simulink model "modelofisicocompletoo"  (R2020a)
settings: Solver=FixedStepAuto  StartTime=0.0  StopTime=inf  FixedStep=0.5e-3  MaxStep=1e-3  RelTol=1e-3
PreLoadFcn:
  | Boat_State = Simulink.Signal;
  | Boat_State.DataType = 'double';
  | Boat_State.SamplingMode = 'Sample based';
  | Boat_State.InitialValue = '[6; 5; 10; 6;  3; 4]';
  | Boat_State.StorageClass = 'ExportedGlobal';
  | Boat_State.Complexity = 'real';
  | Boat_State.Description = 'dsm_description';
undefined symbols (not defined in the file): bac, baiz, bcx, bcy, Beqtran, Bheqd, bw, DiscIntNeverNeededParam, g, Kcy, ksac, ksaiz, ksiac, ksiaiz, Kw, lh0, Meq, Mheq, Rd, Rr, rt, rtd, xl0, xt0, yl0, yt0
libraries: simulink x13, powerlib_meascontrol x4, opclib x4, vrlib x2, dspswit3 x1
(part 2 of 2)

== stateflow chart modelofisicocompletoo/Level1 ==
  state EmergencyMode
  state OFF
  state Sim_pulsadorONOFF1
  state Sim_pulsadorONOFF
  state ON
    state Level1
      state Deegre_Balancer [parallel]
        settings: executionOrder=1
        state OFF
          entry: balancer =0
        state Sim_pulsador
        state Sim_pulsador1
        state ON
          entry: balancer =1
        (default) -> ON.Level1.Deegre_Balancer.OFF
        Sim_pulsador -> ON.Level1.Deegre_Balancer.OFF : [balance_switch==0]
        ON.Level1.Deegre_Balancer.OFF -> ON.Level1.Deegre_Balancer.Sim_pulsador1 : [balance_switch==1]
        ON.Level1.Deegre_Balancer.ON -> Sim_pulsador : [balance_switch==1]
        ON.Level1.Deegre_Balancer.Sim_pulsador1 -> ON.Level1.Deegre_Balancer.ON : [balance_switch==0]
      state Operation_mode [parallel]
        settings: executionOrder=2
        state Automatic
          state Waiting_for_mode
          state Double_cycle
            entry: flag_semiauto = 1;
            flag_end_traj=0;
            flag_send_traj = 0;
            reset_going=0;
            reset_down=0;
            mode_balance = 1;
            state To_boat
              entry:  [vyt,vxt,xend,vx_end,vy_end,len,len2,nx_state] = gen_traj_boat(Boat_State,xl0,yl0,container_x_position,Load_state,Total_mass);
              vx_t=vxt; vy_t=vyt;vxend_t=vx_end;vyend_t=vy_end;len_out=len;len_out2 = len2;Boat_State=nx_state;
              state Go
                entry:
                flag_send_traj = 1;
                reset_going=1;
              state Go_down
                entry:
                flag_send_traj = 1;
                flag_end_traj =1;
                reset_down =1;
              state Finished
                entry:
                flag_end_traj=0;
                flag_send_traj = 0;
              (default) -> ON.Level1.Operation_mode.Automatic.Double_cycle.To_boat.Go
              ON.Level1.Operation_mode.Automatic.Double_cycle.To_boat.Go_down -> ON.Level1.Operation_mode.Automatic.Double_cycle.To_boat.Finished : [flag_finished_taj==1]
              ON.Level1.Operation_mode.Automatic.Double_cycle.To_boat.Go -> ON.Level1.Operation_mode.Automatic.Double_cycle.To_boat.Go_down : [(abs(xend-xl0) <= 0.05) && (theta_amp <= 0.5)]
            state container_to_container
              entry: mode_balance=1;
              [vyt,vxt,xend,vx_end,vy_end,len,len2,nx_state] = gen_traj_cont_cont(Boat_State,xl0,yl0,container_x_position,Load_state,Total_mass);
              vx_t=vxt; vy_t=vyt;vxend_t=vx_end;vyend_t=vy_end;len_out=len;len_out2 = len2;Boat_State=nx_state;
              state Go_down
                entry:
                flag_send_traj = 1;
                flag_end_traj=1;
                reset_down =0;
              state Go
                entry:
                flag_send_traj = 1;
                reset_going=0;
              state Finished1
                entry:
                flag_end_traj=0;
                flag_send_traj = 0;
              (default) -> ON.Level1.Operation_mode.Automatic.Double_cycle.container_to_container.Go
              ON.Level1.Operation_mode.Automatic.Double_cycle.container_to_container.Go -> ON.Level1.Operation_mode.Automatic.Double_cycle.container_to_container.Go_down : [(abs(xend-xl0) <= 0.001) && (theta_amp <= 0.5)]
              ON.Level1.Operation_mode.Automatic.Double_cycle.container_to_container.Go_down -> Finished1 : [flag_finished_taj==1]
            state To_dock
              entry:mode_balance=0;
              [vyt,vxt,xend,vx_end,vy_end,len,len2,nx_state] = gen_traj_dock(Boat_State,xl0,yl0,1,Load_state,Total_mass);
              vx_t=vxt; vy_t=vyt;vxend_t=vx_end;vyend_t=vy_end; len_out=len; len_out2 = len2;Boat_State=nx_state;
              state Go_down
                entry:
                flag_send_traj = 1;
                flag_end_traj=1;
                reset_down =1;
              state Go
                entry:
                flag_send_traj = 1;
                reset_going=1;
              state Finished
                entry:
                flag_semiauto=0;
              (default) -> ON.Level1.Operation_mode.Automatic.Double_cycle.To_dock.Go
              ON.Level1.Operation_mode.Automatic.Double_cycle.To_dock.Go -> ON.Level1.Operation_mode.Automatic.Double_cycle.To_dock.Go_down : [(abs(xend-xl0) <= 1.5) && (theta_amp <= 1.0)]
              ON.Level1.Operation_mode.Automatic.Double_cycle.To_dock.Go_down -> ON.Level1.Operation_mode.Automatic.Double_cycle.To_dock.Finished : [flag_finished_taj==1]
            (default) -> ON.Level1.Operation_mode.Automatic.Double_cycle.To_boat
            ON.Level1.Operation_mode.Automatic.Double_cycle.To_boat.Finished -> container_to_container
            Finished1 -> ON.Level1.Operation_mode.Automatic.Double_cycle.To_dock
          state Simple_cycle
            entry: flag_semiauto = 1;
            flag_end_traj=0;
            flag_send_traj = 0;
            mode_balance = 1;
            state To_boat
              entry: flag_gen_traj = 1;
              [vyt,vxt,xend,vx_end,vy_end,len,len2,nx_state] = gen_traj_boat(Boat_State,xl0,yl0,container_x_position,Load_state,Total_mass);
              vx_t=vxt; vy_t=vyt;vxend_t=vx_end;vyend_t=vy_end;len_out=len;len_out2 = len2;Boat_State=nx_state;
              state Go
                entry:
                flag_send_traj = 1;
                reset_going =0;
              state Go_down
                entry:
                flag_send_traj = 1;
                flag_end_traj =1;
                reset_down=0;
              state Finished
                entry:
                flag_end_traj=0;
                flag_send_traj = 0;
              (default) -> ON.Level1.Operation_mode.Automatic.Simple_cycle.To_boat.Go
              ON.Level1.Operation_mode.Automatic.Simple_cycle.To_boat.Go_down -> ON.Level1.Operation_mode.Automatic.Simple_cycle.To_boat.Finished : [flag_finished_taj==1]
              ON.Level1.Operation_mode.Automatic.Simple_cycle.To_boat.Go -> ON.Level1.Operation_mode.Automatic.Simple_cycle.To_boat.Go_down : [(abs(xend-xl0) <= 0.05) && (theta_amp <= 0.5)]
            state To_dock
              entry:mode_balance=1;
              [vyt,vxt,xend,vx_end,vy_end,len,len2,nx_state] = gen_traj_dock(Boat_State,xl0,yl0,1,Load_state,Total_mass);
              vx_t=vxt; vy_t=vyt;vxend_t=vx_end;vyend_t=vy_end; len_out=len; len_out2 = len2;Boat_State=nx_state;
              state Go_down
                entry:
                flag_send_traj = 1;
                flag_end_traj=1;
                reset_down =1;
              state Go
                entry:
                flag_send_traj = 1;
                reset_going=1;
              state Finished
                entry:
                flag_semiauto=0;
              (default) -> ON.Level1.Operation_mode.Automatic.Simple_cycle.To_dock.Go
              ON.Level1.Operation_mode.Automatic.Simple_cycle.To_dock.Go -> ON.Level1.Operation_mode.Automatic.Simple_cycle.To_dock.Go_down : [(abs(xend-xl0) <= 0.001) && (theta_amp <= 1.0)]
              ON.Level1.Operation_mode.Automatic.Simple_cycle.To_dock.Go_down -> ON.Level1.Operation_mode.Automatic.Simple_cycle.To_dock.Finished : [flag_finished_taj==1]
            (default) -> ON.Level1.Operation_mode.Automatic.Simple_cycle.To_boat
          (default) -> Waiting_for_mode
          Waiting_for_mode -> Double_cycle [order 1] : [Automatic_mode==1]
          Waiting_for_mode -> Simple_cycle [order 2] : [Automatic_mode==0]
        state Manual
          entry:
          flag_semiauto = 0;
          limit_going_down=0;
          limit_vxt_down=0;
          state Operator_handling_load
            state Taking_down
              entry: limit_vxt_down=1;
              state On_air
              state Contact_floor
                entry: limit_going_down =1;
                mode_balance = 0;
              (default) -> ON.Level1.Operation_mode.Manual.Operator_handling_load.Taking_down.On_air
              ON.Level1.Operation_mode.Manual.Operator_handling_load.Taking_down.On_air -> ON.Level1.Operation_mode.Manual.Operator_handling_load.Taking_down.Contact_floor : [Fw<=0.0001]
            state Taking_off
              state On_floor
              state On_air
                entry: limit_going_down =0;
                exit:limit_vxt_down=0;
                mode_balance = 1;
              (default) -> On_floor
              On_floor -> ON.Level1.Operation_mode.Manual.Operator_handling_load.Taking_off.On_air : [Stable_FW_flag]
            (default) -> ON.Level1.Operation_mode.Manual.Operator_handling_load.Taking_down
            ON.Level1.Operation_mode.Manual.Operator_handling_load.Taking_down.Contact_floor -> Taking_off
          state Operator_handling_unload
            entry: limit_vxt_down=1;
            state Taking_down
              state On_air
              state Contact_floor
                entry: limit_going_down =1;
                mode_balance = 0;
              (default) -> ON.Level1.Operation_mode.Manual.Operator_handling_unload.Taking_down.On_air
              ON.Level1.Operation_mode.Manual.Operator_handling_unload.Taking_down.On_air -> ON.Level1.Operation_mode.Manual.Operator_handling_unload.Taking_down.Contact_floor : [Fw<=0.0001]
            state Unloading
              state On_floor_wait_unload
                entry:
                reset_calc_mass =1
              state Transiton
                entry:
                Stable_FW_flag=false
              state On_air
                entry: limit_going_down =0;
                mode_balance = 1;
                exit: limit_vxt_down=0;
              (default) -> On_floor_wait_unload
              On_floor_wait_unload -> Transiton : [Load_state==0]
              Transiton -> ON.Level1.Operation_mode.Manual.Operator_handling_unload.Unloading.On_air : [Stable_FW_flag]
            (default) -> ON.Level1.Operation_mode.Manual.Operator_handling_unload.Taking_down
            ON.Level1.Operation_mode.Manual.Operator_handling_unload.Taking_down.Contact_floor -> Unloading
          (default) -> Operator_handling_load
        state Sim_pulsador_aut
        state Sim_pulsador_man
        (default) -> Manual
        Manual -> Sim_pulsador_aut : [switch_mode==1]
        Sim_pulsador_aut -> Automatic : [switch_mode==0]
        Automatic -> Sim_pulsador_man : [switch_mode==1]
        ON.Level1.Operation_mode.Automatic.Simple_cycle.To_boat.Finished -> Operator_handling_unload : [Automatic_mode==0]
        Sim_pulsador_man -> Manual : [switch_mode==0]
        ON.Level1.Operation_mode.Manual.Operator_handling_unload.Unloading.On_air -> ON.Level1.Operation_mode.Automatic.Simple_cycle.To_dock : [flag_finished_taj==1 && Automatic_mode==0]
      state Load [parallel]
        settings: executionOrder=3
        state not_loaded
          entry: Load_state = 0;
          Total_mass = 15000
          flag_add_random_mass =0;
        state Sim_pulsador2
        state Sim_pulsador1
        state loaded
          entry: Load_state=1;
          flag_add_random_mass =1;
          random_mass = get_rand_mass()
        (default) -> not_loaded
        not_loaded -> ON.Level1.Load.Sim_pulsador1 : [twistlock==1]
        Sim_pulsador2 -> not_loaded : [twistlock==0]
        loaded -> Sim_pulsador2 : [twistlock==1]
        ON.Level1.Load.Sim_pulsador1 -> loaded : [twistlock==0]
  ON -> EmergencyMode [order 2] : [flag_enable_breaks]
  EmergencyMode -> ON : [flag_enable_level1]
  Sim_pulsadorONOFF1 -> OFF : [switch_energy==0]
  OFF -> Sim_pulsadorONOFF : [switch_energy==1]
  ON -> Sim_pulsadorONOFF1 [order 1] : [switch_energy==1]
  (default) -> ON
  Sim_pulsadorONOFF -> ON : [switch_energy==0]
  data: estado_barco function_input; posx_init function_input; posy_init function_input; posx_end function_input; twistlocks function_input; vdyt function_output; vdxt function_output; x_end function_output; vxt_end function_output; vyt_end function_output; ml function_input; lenght function_output; lenght2 function_output; next_state function_output; estado_barco function_input; posx_init function_input; posy_init function_input; posx_end function_input; twistlocks function_input; vdyt function_output; vdxt function_output; x_end function_output; vxt_end function_output; vyt_end function_output; ml function_input; lenght function_output; lenght2 function_output; next_state function_output; estado_barco function_input; posx_init function_input; posy_init function_input; posx_end function_input; twistlocks function_input; vdyt function_output; vdxt function_output; x_end function_output; vxt_end function_output; vyt_end function_output; ml function_input; lenght function_output; lenght2 function_output; next_state function_output; estado_barco function_input; posx_init function_input; posy_init function_input; posx_end function_input; twistlocks function_input; vdyt function_output; vdxt function_output; x_end function_output; vxt_end function_output; vyt_end function_output; ml function_input; lenght function_output; lenght2 function_output; next_state function_output; estado_barco function_input; posx_init function_input; posy_init function_input; posx_end function_input; twistlocks function_input; vdyt function_output; vdxt function_output; x_end function_output; vxt_end function_output; vyt_end function_output; ml function_input; lenght function_output; lenght2 function_output; next_state function_output; rand_mass function_output; xl0 input; switch_mode input; flag_semiauto output; flag_send_traj output; xend local double; flag_end_traj output; vyt local size=20000000,1; vxt local size=20000000,1; vy_end local size=20000000,1; vx_end local size=20000000,1; balance_switch input; switch_energy input; flag_finished_taj input; vyend_t output size=20000000,1; vy_t output size=20000000,1; vxend_t output size=20000000,1; vx_t output size=20000000,1; len_out output; len local; reset_down output; reset_going output; Boat_State data_store_memory; nx_state local double size=6,1 =[0; 0; 0; 0; 0; 0]; len2 local; len_out2 output; limit_vxt_down output; balancer output; mode_balance output; twistlock input; Load_state data_store_memory; limit_going_down output; Stable_FW_flag data_store_memory; Total_mass data_store_memory; container_x_position data_store_memory; flag_add_random_mass output; random_mass output; reset_calc_mass output; flag_enable_level1 input; flag_enable_breaks input; Fw input; theta_amp input; yl0 input; Automatic_mode data_store_memory; flag_gen_traj output
  function [vdyt,vdxt,x_end,vxt_end,vyt_end,lenght,lenght2,next_state] = gen_traj_boat(estado_barco,posx_init,posy_init,posx_end,twistlocks,ml):
    | function [vdyt,vdxt,x_end,vxt_end,vyt_end,lenght,lenght2,next_state] = gen_traj_boat(estado_barco,posx_init,posy_init,posx_end,twistlocks,ml)
    | coder.extrinsic('gen_traj_to_boat');
    | vdyt = [];
    | vdxt = [];
    | vxt_end =[];
    | vyt_end = [];
    | next_state = [0; 0; 0; 0; 0; 0];
    | x_end=0;
    | lenght=0;
    | lenght2=0;
    | coder.varsize('vdyt', [2000000 1]);
    | coder.varsize('vdxt', [2000000 1]);
    | coder.varsize('vyt_end', [2000000 1]);
    | coder.varsize('vxt_end', [2000000 1]);
    | [vdyt,vdxt,x_end,vxt_end,vyt_end,lenght,lenght2,next_state]=gen_traj_to_boat(estado_barco,posx_init,posy_init,posx_end,twistlocks, ml);
    | end
  function [vdyt,vdxt,x_end,vxt_end,vyt_end,lenght,lenght2,next_state] = gen_traj_cont_cont(estado_barco,posx_init,posy_init,posx_end,twistlocks,ml):
    | function [vdyt,vdxt,x_end,vxt_end,vyt_end,lenght,lenght2,next_state] = gen_traj_cont_cont(estado_barco,posx_init,posy_init,posx_end,twistlocks,ml)
    | coder.extrinsic('cont_to_cont');
    | vdyt = [];
    | vdxt = [];
    | vxt_end =[];
    | vyt_end = [];
    | next_state=[0;0;0;0;0;0];
    | x_end=0;
    | lenght = 0;
    | lenght2 = 0;
    | coder.varsize('vdyt', [20000000 1]);
    | coder.varsize('vdxt', [20000000 1]);
    | coder.varsize('vyt_end', [20000000 1]);
    | coder.varsize('vxt_end', [20000000 1]);
    | [vdyt,vdxt,x_end,vxt_end,vyt_end,lenght,lenght2,next_state]=cont_to_cont(estado_barco,posx_init,posy_init,posx_end,twistlocks,ml);
    | end
  function [vdyt,vdxt,x_end,vxt_end,vyt_end,lenght,lenght2,next_state] = gen_traj_dock(estado_barco,posx_init,posy_init,posx_end,twistlocks,ml):
    | function [vdyt,vdxt,x_end,vxt_end,vyt_end,lenght,lenght2,next_state] = gen_traj_dock(estado_barco,posx_init,posy_init,posx_end,twistlocks,ml)
    | coder.extrinsic('gen_traj_to_dock');
    | vdyt = [];
    | vdxt = [];
    | vxt_end =[];
    | vyt_end = [];
    | x_end=0;
    | lenght=0;
    | lenght2 = 0;
    | next_state = [0;0;0;0;0;0];
    | coder.varsize('vdyt', [2000000 1]);
    | coder.varsize('vdxt', [2000000 1]);
    | coder.varsize('vyt_end', [2000000 1]);
    | coder.varsize('vxt_end', [2000000 1]);
    | [vdyt,vdxt,x_end,vxt_end,vyt_end,lenght,lenght2,next_state]=gen_traj_to_dock(estado_barco,posx_init,posy_init,posx_end,twistlocks,ml);
    | end
  function [vdyt,vdxt,x_end,vxt_end,vyt_end,lenght,lenght2,next_state] = gen_traj_boat(estado_barco,posx_init,posy_init,posx_end,twistlocks,ml):
    | function [vdyt,vdxt,x_end,vxt_end,vyt_end,lenght,lenght2,next_state] = gen_traj_boat(estado_barco,posx_init,posy_init,posx_end,twistlocks,ml)
    | coder.extrinsic('gen_traj_to_boat');
    | vdyt = [];
    | vdxt = [];
    | vxt_end =[];
    | vyt_end = [];
    | next_state = [0; 0; 0; 0; 0; 0];
    | x_end=0;
    | lenght=0;
    | lenght2=0;
    | coder.varsize('vdyt', [20000000 1]);
    | coder.varsize('vdxt', [20000000 1]);
    | coder.varsize('vyt_end', [20000000 1]);
    | coder.varsize('vxt_end', [20000000 1]);
    | [vdyt,vdxt,x_end,vxt_end,vyt_end,lenght,lenght2,next_state]=gen_traj_to_boat(estado_barco,posx_init,posy_init,posx_end,twistlocks, ml);
    | end
  function [vdyt,vdxt,x_end,vxt_end,vyt_end,lenght,lenght2,next_state] = gen_traj_dock(estado_barco,posx_init,posy_init,posx_end,twistlocks,ml):
    | function [vdyt,vdxt,x_end,vxt_end,vyt_end,lenght,lenght2,next_state] = gen_traj_dock(estado_barco,posx_init,posy_init,posx_end,twistlocks,ml)
    | coder.extrinsic('gen_traj_to_dock');
    | vdyt = [];
    | vdxt = [];
    | vxt_end =[];
    | vyt_end = [];
    | x_end=0;
    | lenght=0;
    | lenght2 = 0;
    | next_state = [0;0;0;0;0;0];
    | coder.varsize('vdyt', [20000000 1]);
    | coder.varsize('vdxt', [20000000 1]);
    | coder.varsize('vyt_end', [20000000 1]);
    | coder.varsize('vxt_end', [20000000 1]);
    | [vdyt,vdxt,x_end,vxt_end,vyt_end,lenght,lenght2,next_state]=gen_traj_to_dock(estado_barco,posx_init,posy_init,posx_end,twistlocks,ml);
    | end
  function rand_mass  = get_rand_mass:
    | function rand_mass  = get_rand_mass()
    | rand_mass = (randi(10000) + 2000);
    | end

== matlab function modelofisicocompletoo/sending_setpoint_mechanisim/Trajectoria vxt/Subsystem3/Resettable Subsystem/MATLAB Function ==
  data: len_vec input; qd input size=20000000,1; cont_i input; cont output; vt output
 function [cont, vt] = fcn(len_vec, qd,cont_i)
 if (cont_i<len_vec)
   cont=cont_i+1;
   vt = qd(cont,1);
 else
  vt = 0;
  cont=inf;
 end
 end

== matlab function modelofisicocompletoo/sending_setpoint_mechanisim/Trajectoria vyt/Subsystem3/Resettable Subsystem/MATLAB Function ==
  data: len_vec input; qd input size=20000000,1; cont_i input; cont output; vt output
 function [cont, vt] = fcn(len_vec, qd,cont_i)
 if (cont_i<len_vec)
   cont=cont_i+1;
   vt = qd(cont,1);
 else
  vt = 0;
  cont=inf;
 end
 end

== matlab function modelofisicocompletoo/sending_setpoint_mechanisim/Trajectoria vyt1/Subsystem3/Resettable Subsystem/MATLAB Function ==
  data: len_vec input; qd input size=20000000,1; cont_i input; cont output; vt output
 function [cont, vt] = fcn(len_vec, qd,cont_i)
 if (cont_i<len_vec)
   cont=cont_i+1;
   vt = qd(cont,1);
 else
  vt = 0;
  cont=inf;
 end
 end

== matlab function modelofisicocompletoo/sending_setpoint_mechanisim/Trajectoria vyt3/Subsystem3/Resettable Subsystem/MATLAB Function ==
  data: len_vec input; qd input size=20000000,1; cont_i input; cont output; vt output
 function [cont, vt] = fcn(len_vec, qd,cont_i)
 if (cont_i<len_vec)
   cont=cont_i+1;
   vt = qd(cont,1);
 else
  vt = 0;
  cont=inf;
 end
 end
